simulink model "CSTR_jacket"  (R2024a)
settings: Solver=ode45  StartTime=0.0  StopTime=10.0  MaxStep=0.1  RelTol=1e-3  EnableMultiTasking=on
settings Model: Creator=amankhilani  LastModifiedBy=amankhilani
settings DataIOCC: LimitDataPoints=on  SaveFormat=Structure  SignalLoggingSaveFormat=ModelDataLogs  ReturnWorkspaceOutputs=off
settings OptimizationCC: InitFltsAndDblsToZero=on  LifeSpan=inf
settings DebuggingCC: SaveWithParameterizedLinksMsg=none  UnderspecifiedInitializationDetection=Classic  MergeDetectMultiDrivingBlocksExec=none  SignalResolutionControl=TryResolveAllWithWarning  SolverPrmCheckMsg=warning  MultiTaskDSMMsg=warning  MultiTaskCondExecSysMsg=none  FcnCallInpInsideContextMsg=warning  UnconnectedInputMsg=warning  UnconnectedOutputMsg=warning  UnconnectedLineMsg=warning  SFUnexpectedBacktrackingDiag=warning  SFNoUnconditionalDefaultTransitionDiag=warning  SFExecutionAtInitializationDiag=none  ArithmeticOperatorsInVariantConditions=warning
settings HardwareCC: ProdBitPerPointer=32  ProdBitPerSizeT=32  ProdBitPerPtrDiffT=32  ProdLargestAtomicFloat=None  ProdIntDivRoundTo=Undefined  ProdEndianess=Unspecified  ProdWordSize=32  ProdHWDeviceType=32-bit Generic
settings ModelReferenceCC: PropagateSignalLabelsOutOfModel=off
settings RTWCC: GPUComputeCapability=3.5
settings CodeAppCC: StateflowObjectComments=on
settings GRTTargetCC: TargetFcnLib=ansi_tfl_tmw.mat  TargetLangStandard=C89/C90 (ANSI)  CombineOutputUpdateFcns=off  GRTInterface=on
settings ConfigComp: CovMetricSettings=dw  CovSaveCumulativeToWorkspaceVar=on  CovSaveSingleToWorkspaceVar=on

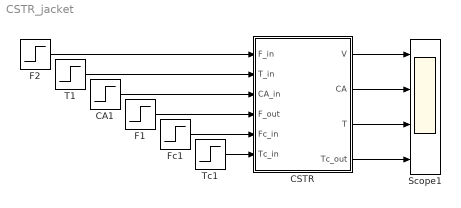
== system CSTR_jacket ==
  CA1 : Step  Before=2  After=2  SampleTime=0
  CSTR : Subsystem  mask(Nonisothermal CSTR){k0=1.2e+10, ER=8100, n=1, dHr=-120e+6, rho=1e+6, Cp=1, rhoc=1e+6, Cpc=1, UA=5e+6, Vc=0.4, Vini=1, Tini=385.69, Tcini=352.59, CAini=0.1983}
      mask prompts: k0 "頻度因子 k0"; ER "活性化エネルギー／気体定数 E/R"; n "反応次数 n"; dHr "反応熱 ΔHr"; rho "流体液密度 ρ"; Cp "流体熱容量 Cp"; rhoc "冷媒液密度 ρc"; Cpc "冷媒熱容量 Cpc"; UA "総括伝熱係数×伝熱面積 UA"; Vc "ジャケット体積 Vc"; Vini "ホールドアップ(V)初期値"; Tini "反応温度(T)初期値"; Tcini "冷媒温度(Tc)初期値"; CAini "反応物濃度(CA)初期値"
      mask help: 非等温完全混合槽型反応器
  F1 : Step  Before=1  SampleTime=0
  F2 : Step  Before=1  SampleTime=0
  Fc1 : Step  Before=6  After=6.6  SampleTime=0
  Scope1 : Scope  NumInputPorts=4
  T1 : Step  Before=335  After=335  SampleTime=0
  Tc1 : Step  Before=325  After=325  SampleTime=0
  wires:
  F2/1 -> CSTR/1(F_in)
  T1/1 -> CSTR/2(T_in)
  CA1/1 -> CSTR/3(CA_in)
  F1/1 -> CSTR/4(F_out)
  Fc1/1 -> CSTR/5(Fc_in)
  Tc1/1 -> CSTR/6(Tc_in)
  CSTR/1(V) -> Scope1/1
  CSTR/2(CA) -> Scope1/2
  CSTR/3(T) -> Scope1/3
  CSTR/4(Tc_out) -> Scope1/4

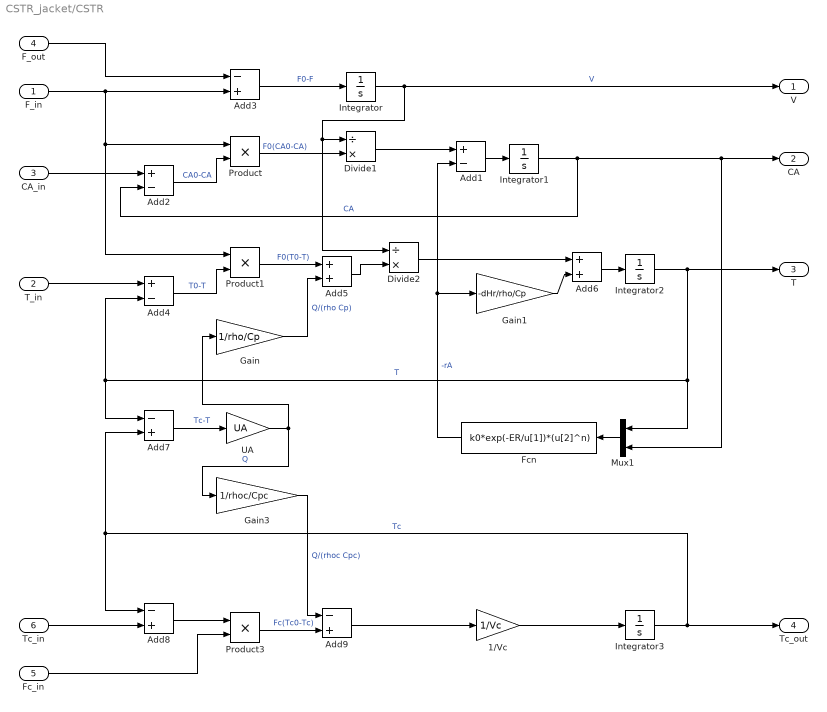
== system CSTR_jacket/CSTR ==
  F_in : Inport
  T_in : Inport  Port=2
  CA_in : Inport  Port=3
  F_out : Inport  Port=4
  Fc_in : Inport  Port=5
  Tc_in : Inport  Port=6
  1/Vc : Gain  Gain=1/Vc
  Add1 : Sum  Inputs=+-
  Add2 : Sum  Inputs=+-
  Add{3,7..9} (4 alike) : Sum  Inputs=-+
  Add4 : Sum  Inputs=+-
  Add5 : Sum
  Add6 : Sum
  Divide1 : Product  Inputs=/*
  Divide2 : Product  Inputs=/*
  Fcn : Fcn  Expr=k0*exp(-ER/u[1])*(u[2]^n)
  Gain : Gain  Gain=1/rho/Cp
  Gain1 : Gain  Gain=-dHr/rho/Cp
  Gain3 : Gain  Gain=1/rhoc/Cpc
  Integrator : Integrator  InitialCondition=Vini
  Integrator1 : Integrator  InitialCondition=CAini
  Integrator2 : Integrator  InitialCondition=Tini
  Integrator3 : Integrator  InitialCondition=Tcini
  Mux1 : Mux  Inputs=2
  Product : Product  RndMeth=Zero
  Product1 : Product  RndMeth=Zero
  Product3 : Product  RndMeth=Zero
  UA : Gain  Gain=UA
  V : Outport
  CA : Outport  Port=2
  T : Outport  Port=3
  Tc_out : Outport  Port=4
  wires:
  Integrator/1 -> Divide1/1, Divide2/1, V/1  "V"
  Add3/1 -> Integrator/1  "F0-F"
  F_in/1 -> Product1/1, Product/1, Add3/2
  F_out/1 -> Add3/1
  Product/1 -> Divide1/2  "F0(CA0-CA)"
  Fcn/1 -> Add1/2, Gain1/1  "-rA"
  CA_in/1 -> Add2/1
  Add2/1 -> Product/2  "CA0-CA"
  Integrator1/1 -> Add2/2, CA/1, Mux1/2  "CA"
  Divide1/1 -> Add1/1
  Add1/1 -> Integrator1/1
  Product1/1 -> Add5/1  "F0(T0-T)"
  Add4/1 -> Product1/2  "T0-T"
  T_in/1 -> Add4/1
  Add5/1 -> Divide2/2
  Gain/1 -> Add5/2  "Q/(rho Cp)"
  Divide2/1 -> Add6/1
  Gain1/1 -> Add6/2
  Integrator2/1 -> T/1, Add4/2, Add7/1, Mux1/1  "T"
  Add6/1 -> Integrator2/1
  Fc_in/1 -> Product3/2
  UA/1 -> Gain/1, Gain3/1  "Q"
  Add7/1 -> UA/1  "Tc-T"
  Mux1/1 -> Fcn/1
  Product3/1 -> Add9/2  "Fc(Tc0-Tc)"
  Add9/1 -> 1/Vc/1
  1/Vc/1 -> Integrator3/1
  Integrator3/1 -> Tc_out/1, Add7/2, Add8/1  "Tc"
  Tc_in/1 -> Add8/2
  Add8/1 -> Product3/1
  Gain3/1 -> Add9/1  "Q/(rhoc Cpc)"
